simulink model "DCMG_BDCUIO_jan2025_scenario_4"  (R2018b)
settings: Solver=ode1  StartTime=0.0  StopTime=2  FixedStep=1e-6  RelTol=1e-3
undefined symbols (not defined in the file): Cdc, Cpv, dEgdT, EgRef, gcbh, k1, KIvp, KPvp, Rsh_array5pc, sigbuilder_block, sps_rtmsupport, Tref_K, Ts, VT_ref
libraries: powerlib x42, spsPVarrayModel x3
(part 1 of 6)
settings Model: Creator=SAID  LastModifiedBy=TRETEC

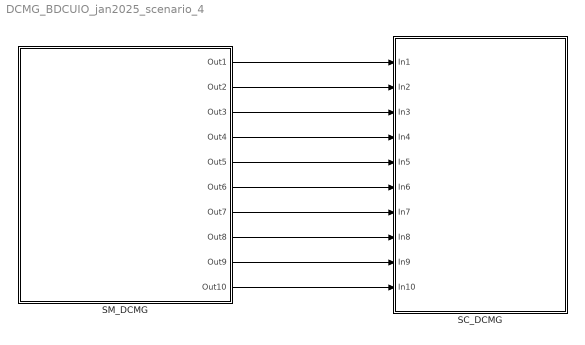
== system DCMG_BDCUIO_jan2025_scenario_4 ==
  SC_DCMG : Subsystem
  SM_DCMG : Subsystem
  wires:
  SM_DCMG/1(Out1) -> SC_DCMG/1(In1)
  SM_DCMG/2(Out2) -> SC_DCMG/2(In2)
  SM_DCMG/3(Out3) -> SC_DCMG/3(In3)
  SM_DCMG/4(Out4) -> SC_DCMG/4(In4)
  SM_DCMG/5(Out5) -> SC_DCMG/5(In5)
  SM_DCMG/6(Out6) -> SC_DCMG/6(In6)
  SM_DCMG/7(Out7) -> SC_DCMG/7(In7)
  SM_DCMG/8(Out8) -> SC_DCMG/8(In8)
  SM_DCMG/9(Out9) -> SC_DCMG/9(In9)
  SM_DCMG/10(Out10) -> SC_DCMG/10(In10)

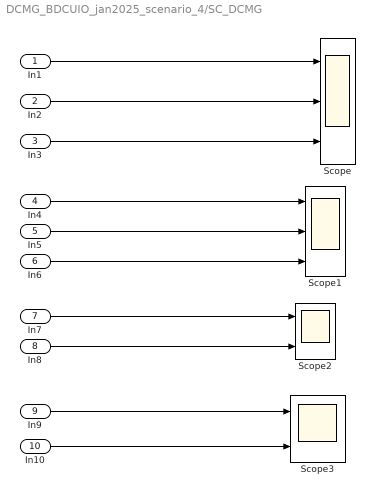
== system DCMG_BDCUIO_jan2025_scenario_4/SC_DCMG ==
  In1 : Inport
  In2 : Inport  Port=2
  In3 : Inport  Port=3
  In4 : Inport  Port=4
  In5 : Inport  Port=5
  In6 : Inport  Port=6
  In7 : Inport  Port=7
  In8 : Inport  Port=8
  In9 : Inport  Port=9
  In10 : Inport  Port=10
  Scope : Scope  NumInputPorts=3
  Scope1 : Scope  NumInputPorts=3
  Scope2 : Scope  NumInputPorts=2
  Scope3 : Scope  NumInputPorts=2
  wires:
  In1/1 -> Scope/1
  In2/1 -> Scope/2
  In3/1 -> Scope/3
  In4/1 -> Scope1/1
  In5/1 -> Scope1/2
  In6/1 -> Scope1/3
  In7/1 -> Scope2/1
  In8/1 -> Scope2/2
  In9/1 -> Scope3/1
  In10/1 -> Scope3/2
